simulink model "Mpc_SimMechanics_with_standing"  (R2017b)
settings: Solver=ode45  StartTime=0  StopTime=10  FixedStep=0.0005  EnableMultiTasking=on
InitFcn:
  | isSim = 1;
  | 
  | PreFunctions.CustomInitFcn_with_standing;
  | PreFunctions.simulationInitFcn_with_standing;
undefined symbols (not defined in the file): alpha_x, alpha_y, DiagnosticCodes, DynamicMatrixLibrary, motorPositions, motorVelocities, pelvisPosition, pelvisVelocity, sample_time, X, Y, Z
libraries: sm_lib x170, nesl_utility x75, Contact_Forces_Lib x6, ComponentLibrary x5, xpcrtudplib x2, slrtlib x1
(part 1 of 8)
settings Model: TunableVars=c_CovPos_abduction,c_CovPos_knee,c_CovPos_qj1,c_CovPos_qj2,c_CovPos_qj3,c_CovPos_rotation,c_CovPos_thigh,c_CovPos_toe,c_CovVel_abduction,c_CovVel_knee,c_CovVel_qj1,c_CovVel_qj2,c_CovVel_qj3,c_CovVel_rotation,c_CovVel_thigh,c_CovVel_toe,c_Cov_AngularVelocity,c_Cov_Euler,c_Cov_Euler_rates,c_Cov_LinearAccelerator_xy,c_Cov_LinearAccelerator_z,c_Cov_Lx_LRToe_stTD0,c_Cov_Ly_LRToe_stTD0,c_Cov_Orientation,c_Cov_rpx_LRToe_body,c_Cov_rpx_LRToe_stTD0,c_Cov_rpy_LRToe_body,c_Cov_rpy_LRToe_stTD0,c_Cov_rpz_LRToe_body,c_H_fil_param,c_IK_max_iter_num,c_Kd_abduction,c_Kd_knee,c_Kd_pitch,c_Kd_roll,c_Kd_rotation,c_Kd_st_rotation,c_Kd_thigh,c_Kd_toe,c_Kd_yaw,c_Kp_abduction,c_Kp_knee,c_Kp_pitch,c_Kp_roll,c_Kp_rotation,c_Kp_st_rotation,c_Kp_thigh,c_Kp_toe,c_Kp_yaw,c_KsL_1,c_KsL_2,c_KsR_1,c_KsR_2,c_Tx_slide_toe_2,c_Ty_slide_toe_2,c_Tz_slide_toe_2,c_Vx_tgd_fil_param,c_Vx_tgd_offset,c_Vy_tgd_avg_fil_param,c_Vy_tgd_offset,c_adjusted_desired_roll_angle_fil_param,c_com_x_offset,c_desired_com2stToe_lateral_fil_param,c_dop,c_history_length,c_knee_cp_time,c_lateral_correction_gain,c_max_st_rotation_motor_torque,c_max_turn_per_sec,c_one_step_max_vel_gain,c_rp_LRToe_fil_param,c_st_rotation_torque_ramp_time,c_stance_thre_lb,c_stance_thre_lb_2,c_stance_thre_ub,c_stance_thre_ub_2,c_toe_leave_ground_lb,c_toe_leave_ground_ub,c_torque_transition_time,c_u_abduction_swing_cp,c_u_knee_cp,c_u_pitch_cp,c_u_roll_cp,c_use_dq_AR_for_PD,c_vx_slide_toe_1,c_vx_slide_toe_2,c_vy_slide_toe_1,c_vy_slide_toe_2,c_vz_slide_toe_1,c_vz_slide_toe_2,c_yaw_error_fil_param  TunableVarsStorageClass=Auto,Auto,Auto,Auto,Auto,Auto,Auto,Auto,Auto,Auto,Auto,Auto,Auto,Auto,Auto,Auto,Auto,Auto,Auto,Auto,Auto,Auto,Auto,Auto,Auto,Auto,Auto,Auto,Auto,Auto,Auto,Auto,Auto,Auto,Auto,Auto,Auto,Auto,Auto,Auto,Auto,Auto,Auto,Auto,Auto,Auto,Auto,Auto,Auto,Auto,Auto,Auto,Auto,Auto,Auto,Auto,Auto,Auto,Auto,Auto,Auto,Auto,Auto,Auto,Auto,Auto,Auto,Auto,Auto,Auto,Auto,Auto,Auto,Auto,Auto,Auto,Auto,Auto,Auto,Auto,Auto,Auto,Auto,Auto,Auto,Auto,Auto,Auto,Auto,Auto,Auto  TunableVarsTypeQualifier=,,,,,,,,,,,,,,,,,,,,,,,,,,,,,,,,,,,,,,,,,,,,,,,,,,,,,,,,,,,,,,,,,,,,,,,,,,,,,,,,,,,,,,,,,,  Creator=case  LastModifiedBy=gibso
settings SolverCC: ZeroCrossControl=DisableAll  InsertRTBMode=Always
settings DataIOCC: SaveOutput=off  SignalLogging=off  DSMLogging=off  SaveTime=off
settings OptimizationCC: UseFloatMulNetSlope=on  EfficientFloat2IntCast=on  LifeSpan=inf  SimCompilerOptimization=on  AccelVerboseBuild=on
settings DebuggingCC: ReadBeforeWriteMsg=DisableAll  WriteAfterWriteMsg=DisableAll  WriteAfterReadMsg=DisableAll  ParameterUnderflowMsg=error  ParameterTunabilityLossMsg=error  UniqueDataStoreMsg=error  AllowSymbolicDim=off  StrictBusMsg=ErrorOnBusTreatedAsVector  SFUnexpectedBacktrackingDiag=warning  SFNoUnconditionalDefaultTransitionDiag=warning  SFExecutionAtInitializationDiag=none
settings HardwareCC: TargetBitPerPointer=64  TargetBitPerSizeT=64  TargetBitPerPtrDiffT=64  TargetLongLongMode=on  TargetIntDivRoundTo=Zero  TargetEndianess=LittleEndian  TargetWordSize=64  TargetHWDeviceType=MATLAB Host  ProdEqTarget=off
settings ModelReferenceCC: EnableParallelModelReferenceBuilds=on  ModelReferenceNumInstancesAllowed=Zero  ModelReferenceMinAlgLoopOccurrences=on  PropagateSignalLabelsOutOfModel=off
settings SFSimCC: SimUserIncludeDirs=$root_dir$\CustomCodes\utils\funcs\KinDyn200511_221619
settings SFSimCC: SimUserSources=|
  | R_LeftAbductionJoint_src.c
  | R_LeftThighJoint_src.c
  | R_RightAbductionJoint_src.c
  | R_RightThighJoint_src.c
  | 
  | AMworld_about_pA_src.c
  | 
  | Jb_BasePosX_src.c
  | Jb_BasePosY_src.c
  | Jb_BasePosZ_src.c
  | Jb_BaseRotX_src.c
  | Jb_BaseRotY_src.c
  | Jb_BaseRotZ_src.c
  | Jb_LeftAbductionJoint_src.c
  | Jb_LeftAnkleJoint_src.c
  | Jb_LeftHip_src.c
  | Jb_LeftKneeJoint_src.c
  | Jb_LeftKneeSpringJoint_src.c
  | Jb_LeftKnee_src.c
  | Jb_LeftPelvisRotation_src.c
  | Jb_LeftRotationJoint_src.c
  | Jb_LeftShin_src.c
  | Jb_LeftTarsus_src.c
  | Jb_LeftThighJoint_src.c
  | Jb_LeftThigh_src.c
  | Jb_LeftToeBottomBack_src.c
  | Jb_LeftToeBottomFront_src.c
  | Jb_LeftToeBottom_src.c
  | Jb_LeftToeJoint_src.c
  | Jb_LeftToe_src.c
  | Jb_Pelvis_src.c
  | Jb_RightAbductionJoint_src.c
  | Jb_RightAnkleJoint_src.c
  | Jb_RightHip_src.c
  | Jb_RightKneeJoint_src.c
  | Jb_RightKneeSpringJoint_src.c
  | Jb_RightKnee_src.c
  | Jb_RightPelvisRotation_src.c
  | Jb_RightRotationJoint_src.c
  | Jb_RightShin_src.c
  | Jb_RightTarsus_src.c
  | Jb_RightThighJoint_src.c
  | Jb_RightThigh_src.c
  | Jb_RightToeBottomBack_src.c
  | Jb_RightToeBottomFront_src.c
  | Jb_RightToeBottom_src.c
  | Jb_RightToeJoint_src.c
  | Jb_RightToe_src.c
  | 
  | Jdq_AMworld_about_pA_src.c
  | 
  | 
  | Jp_COM_src.c
  | Jp_LeftAbductionJoint_src.c
  | Jp_LeftAnkleJoint_src.c
  | Jp_LeftHip_src.c
  | Jp_LeftKneeJoint_src.c
  | Jp_LeftKneeSpringJoint_src.c
  | Jp_LeftKnee_src.c
  | Jp_LeftPelvisRotation_src.c
  | Jp_LeftRotationJoint_src.c
  | Jp_LeftShin_src.c
  | Jp_LeftTarsus_src.c
  | Jp_LeftThighJoint_src.c
  | Jp_LeftThigh_src.c
  | Jp_LeftToeBottomBack_src.c
  | Jp_LeftToeBottomFront_src.c
  | Jp_LeftToeBottom_src.c
  | Jp_LeftToeJoint_src.c
  | Jp_LeftToe_src.c
  | Jp_Pelvis_src.c
  | Jp_RightAbductionJoint_src.c
  | Jp_RightAnkleJoint_src.c
  | Jp_RightHip_src.c
  | Jp_RightKneeJoint_src.c
  | Jp_RightKneeSpringJoint_src.c
  | Jp_RightKnee_src.c
  | Jp_RightPelvisRotation_src.c
  | Jp_RightRotationJoint_src.c
  | Jp_RightShin_src.c
  | Jp_RightTarsus_src.c
  | Jp_RightThighJoint_src.c
  | Jp_RightThigh_src.c
  | Jp_RightToeBottomBack_src.c
  | Jp_RightToeBottomFront_src.c
  | Jp_RightToeBottom_src.c
  | Jp_RightToeJoint_src.c
  | Jp_RightToe_src.c
  | 
  | p_BasePosX_src.c
  | p_BasePosY_src.c
  | p_BasePosZ_src.c
  | p_BaseRotX_src.c
  | p_BaseRotY_src.c
  | p_BaseRotZ_src.c
  | p_COM_src.c
  | p_LeftAbductionJoint_src.c
  | p_LeftAnkleJoint_src.c
  | p_LeftHip_src.c
  | p_LeftKneeJoint_src.c
  | p_LeftKneeSpringJoint_src.c
  | p_LeftKnee_src.c
  | p_LeftPelvisRotation_src.c
  | p_LeftRotationJoint_src.c
  | p_LeftShin_src.c
  | p_LeftTarsus_src.c
  | p_LeftThighJoint_src.c
  | p_LeftThigh_src.c
  | p_LeftToeBottomBack_src.c
  | p_LeftToeBottomFront_src.c
  | p_LeftToeBottom_src.c
  | p_LeftToeJoint_src.c
  | p_LeftToe_src.c
  | p_Pelvis_src.c
  | p_RightAbductionJoint_src.c
  | p_RightAnkleJoint_src.c
  | p_RightHip_src.c
  | p_RightKneeJoint_src.c
  | p_RightKneeSpringJoint_src.c
  | p_RightKnee_src.c
  | p_RightPelvisRotation_src.c
  | p_RightRotationJoint_src.c
  | p_RightShin_src.c
  | p_RightTarsus_src.c
  | p_RightThighJoint_src.c
  | p_RightThigh_src.c
  | p_RightToeBottomBack_src.c
  | p_RightToeBottomFront_src.c
  | p_RightToeBottom_src.c
  | p_RightToeJoint_src.c
  | p_RightToe_src.c
  | 
  | T_LeftToeBottomBack_src.c
  | T_LeftToeBottomFront_src.c
  | T_LeftToeBottom_src.c
  | T_RightToeBottomBack_src.c
  | T_RightToeBottomFront_src.c
  | T_RightToeBottom_src.c
  | 
  | J_LL_Left_src.c
  | J_LL_Right_src.c
  | LL_Left_src.c
  | LL_Right_src.c
settings RTWCC: Description=Generic Real-Time Target  RTWUseSimCustomCode=on  CustomInclude=$root_dir$\CustomCodes\utils\funcs\KinDyn200511_221619  BuildConfiguration=Faster Runs  CheckMdlBeforeBuild=Warning
settings RTWCC: CustomSource=|
  | R_LeftAbductionJoint_src.c
  | R_LeftThighJoint_src.c
  | R_RightAbductionJoint_src.c
  | R_RightThighJoint_src.c
  | 
  | AMworld_about_pA_src.c
  | 
  | Jb_BasePosX_src.c
  | Jb_BasePosY_src.c
  | Jb_BasePosZ_src.c
  | Jb_BaseRotX_src.c
  | Jb_BaseRotY_src.c
  | Jb_BaseRotZ_src.c
  | Jb_LeftAbductionJoint_src.c
  | Jb_LeftAnkleJoint_src.c
  | Jb_LeftHip_src.c
  | Jb_LeftKneeJoint_src.c
  | Jb_LeftKneeSpringJoint_src.c
  | Jb_LeftKnee_src.c
  | Jb_LeftPelvisRotation_src.c
  | Jb_LeftRotationJoint_src.c
  | Jb_LeftShin_src.c
  | Jb_LeftTarsus_src.c
  | Jb_LeftThighJoint_src.c
  | Jb_LeftThigh_src.c
  | Jb_LeftToeBottomBack_src.c
  | Jb_LeftToeBottomFront_src.c
  | Jb_LeftToeBottom_src.c
  | Jb_LeftToeJoint_src.c
  | Jb_LeftToe_src.c
  | Jb_Pelvis_src.c
  | Jb_RightAbductionJoint_src.c
  | Jb_RightAnkleJoint_src.c
  | Jb_RightHip_src.c
  | Jb_RightKneeJoint_src.c
  | Jb_RightKneeSpringJoint_src.c
  | Jb_RightKnee_src.c
  | Jb_RightPelvisRotation_src.c
  | Jb_RightRotationJoint_src.c
  | Jb_RightShin_src.c
  | Jb_RightTarsus_src.c
  | Jb_RightThighJoint_src.c
  | Jb_RightThigh_src.c
  | Jb_RightToeBottomBack_src.c
  | Jb_RightToeBottomFront_src.c
  | Jb_RightToeBottom_src.c
  | Jb_RightToeJoint_src.c
  | Jb_RightToe_src.c
  | 
  | Jdq_AMworld_about_pA_src.c
  | 
  | 
  | Jp_COM_src.c
  | Jp_LeftAbductionJoint_src.c
  | Jp_LeftAnkleJoint_src.c
  | Jp_LeftHip_src.c
  | Jp_LeftKneeJoint_src.c
  | Jp_LeftKneeSpringJoint_src.c
  | Jp_LeftKnee_src.c
  | Jp_LeftPelvisRotation_src.c
  | Jp_LeftRotationJoint_src.c
  | Jp_LeftShin_src.c
  | Jp_LeftTarsus_src.c
  | Jp_LeftThighJoint_src.c
  | Jp_LeftThigh_src.c
  | Jp_LeftToeBottomBack_src.c
  | Jp_LeftToeBottomFront_src.c
  | Jp_LeftToeBottom_src.c
  | Jp_LeftToeJoint_src.c
  | Jp_LeftToe_src.c
  | Jp_Pelvis_src.c
  | Jp_RightAbductionJoint_src.c
  | Jp_RightAnkleJoint_src.c
  | Jp_RightHip_src.c
  | Jp_RightKneeJoint_src.c
  | Jp_RightKneeSpringJoint_src.c
  | Jp_RightKnee_src.c
  | Jp_RightPelvisRotation_src.c
  | Jp_RightRotationJoint_src.c
  | Jp_RightShin_src.c
  | Jp_RightTarsus_src.c
  | Jp_RightThighJoint_src.c
  | Jp_RightThigh_src.c
  | Jp_RightToeBottomBack_src.c
  | Jp_RightToeBottomFront_src.c
  | Jp_RightToeBottom_src.c
  | Jp_RightToeJoint_src.c
  | Jp_RightToe_src.c
  | 
  | p_BasePosX_src.c
  | p_BasePosY_src.c
  | p_BasePosZ_src.c
  | p_BaseRotX_src.c
  | p_BaseRotY_src.c
  | p_BaseRotZ_src.c
  | p_COM_src.c
  | p_LeftAbductionJoint_src.c
  | p_LeftAnkleJoint_src.c
  | p_LeftHip_src.c
  | p_LeftKneeJoint_src.c
  | p_LeftKneeSpringJoint_src.c
  | p_LeftKnee_src.c
  | p_LeftPelvisRotation_src.c
  | p_LeftRotationJoint_src.c
  | p_LeftShin_src.c
  | p_LeftTarsus_src.c
  | p_LeftThighJoint_src.c
  | p_LeftThigh_src.c
  | p_LeftToeBottomBack_src.c
  | p_LeftToeBottomFront_src.c
  | p_LeftToeBottom_src.c
  | p_LeftToeJoint_src.c
  | p_LeftToe_src.c
  | p_Pelvis_src.c
  | p_RightAbductionJoint_src.c
  | p_RightAnkleJoint_src.c
  | p_RightHip_src.c
  | p_RightKneeJoint_src.c
  | p_RightKneeSpringJoint_src.c
  | p_RightKnee_src.c
  | p_RightPelvisRotation_src.c
  | p_RightRotationJoint_src.c
  | p_RightShin_src.c
  | p_RightTarsus_src.c
  | p_RightThighJoint_src.c
  | p_RightThigh_src.c
  | p_RightToeBottomBack_src.c
  | p_RightToeBottomFront_src.c
  | p_RightToeBottom_src.c
  | p_RightToeJoint_src.c
  | p_RightToe_src.c
  | 
  | T_LeftToeBottomBack_src.c
  | T_LeftToeBottomFront_src.c
  | T_LeftToeBottom_src.c
  | T_RightToeBottomBack_src.c
  | T_RightToeBottomFront_src.c
  | T_RightToeBottom_src.c
  | 
  | J_LL_Left_src.c
  | J_LL_Right_src.c
  | LL_Left_src.c
  | LL_Right_src.c
settings CodeAppCC: GenerateComments=off  SimulinkBlockComments=off
settings GRTTargetCC: MatFileLogging=off  MultiInstanceERTCode=on  CodeInterfacePackaging=Reusable function  SupportNonFinite=off  GenerateAllocFcn=on
settings ConfigComp: CovMetricSettings=dw  CovHtmlReporting=on  CovSaveCumulativeToWorkspaceVar=on  CovSaveSingleToWorkspaceVar=on  CovExternalEMLEnable=off
settings SimscapeCC: SimscapeNormalizeSystem=off
settings DiagnosticsConfigSet: SimMechanicsRigidlyBoundBlock=warning
settings ExplorerConfigSet: InternalSimMechanicsExplorerSettings="<ExplorerConfiguration><canonicalview>default</canonicalview><AnimationSetting><BasePlaybackSpeed>1.0</BasePlaybackSpeed><PlaybackSpeedFactor>1.0</PlaybackSpeedFactor></AnimationSetting><TilePanel><TileInfo><Tiles Columns=\"1\" Count=\"2\" Rows=\"2\"><Column Weight=\"1\"/><Row Weight=\"0.4993\"/><Row Weight=\"0.5007\"/><Tile Height=\"1\" Width=\"1\" X=\"0\" Y=\"0\"/><Tile Height=\"1\" Width=\"1\" X=\"0\" Y=\"1\"/></Tiles></TileInfo><SceneInfo><SceneViewer><BGColor><R>0.60000002384185791</R><G>0.60000002384185791</G><B>0.60000002384185791</B></BGColor><Camera><DoPerspective>off</DoPerspective><Position><X>35.4589435267912592</X><Y>10.7098035623800421</Y><Z>2.09856989778365666</Z></Position><Center><X>1.22559782766984426e-06</X><Y>10.7098035623800421</Y><Z>2.09856989778365666</Z></Center><Up><X>-0</X><Y>0</Y><Z>1</Z></Up><ViewLimDist>1</ViewLimDist><YLim>6.75206365413680487</YLim><XLim>15.8384121715609041</XLim></Camera></SceneViewer><SceneViewer><BGColor><R>0.60000002384185791</R><G>0.60000002384185791</G><B>0.60000002384185791</B></BGColor><Camera><DoPerspective>off</DoPerspective><Position><X>-0.287232906465883953</X><Y>-35.4589435232020875</Y><Z>0.354651545256036704</Z></Position><Center><X>-0.287232906465883953</X><Y>3.60980493385731904e-07</Y><Z>0.354651545256036704</Z></Center><Up><X>0</X><Y>-0</Y><Z>1</Z></Up><ViewLimDist>1</ViewLimDist><YLim>2.45492732079823162</YLim><XLim>5.74215193839130489</XLim></Camera></SceneViewer></SceneInfo></TilePanel><MechEditorPanel><Cameras><Camera><Id>Camera1</Id><Value><Name>Tracking Camera</Name><NativeCamera><PositionTrackingFeature>Cassie.Cassie_Simulation.World.Tracking_Camera.F</PositionTrackingFeature><CenterTrackingFeature>Cassie.Cassie_Simulation.World.Tracking_Camera_Target.F</CenterTrackingFeature><UpVectorTrackingFeature>Cassie.Cassie_Simulation.World.Tracking_Camera_Target.F</UpVectorTrackingFeature><CenterTrackingOrigin>on</CenterTrackingOrigin><UpVectorTrackingDirection>+Z</UpVectorTrackingDirection></NativeCamera></Value></Camera><Camera><Id>Camera2</Id><Value><Name>Fixed Camera</Name><NativeCamera><PositionTrackingFeature>Cassie.Cassie_Simulation.World.Fixed_Camera.F</PositionTrackingFeature><CenterTrackingFeature>Cassie.Cassie_Simulation.World.Fixed_Camera_Target.F</CenterTrackingFeature><UpVectorTrackingFeature>Cassie.Cassie_Simulation.World.Fixed_Camera_Target.F</UpVectorTrackingFeature><CenterTrackingOrigin>on</CenterTrackingOrigin><UpVectorTrackingDirection>+Z</UpVectorTrackingDirection></NativeCamera></Value></Camera><Camera><Id>Camera3</Id><Value><Name>tracking camera positive y</Name><NativeCamera><PositionTrackingFeature>Cassie.Cassie_Simulation.Cassie_Pelvis_World</PositionTrackingFeature><CenterTrackingFeature/><UpVectorTrackingFeature/><CenterTrackingOrigin>off</CenterTrackingOrigin><CenterTrackingDirection>+Y</CenterTrackingDirection><UpVectorTrackingDirection>+Z</UpVectorTrackingDirection></NativeCamera></Value></Camera></Cameras><GfxPanelCameraMap/><VideoCreator><PlaybackSpeedRatio>1.0</PlaybackSpeedRatio><FrameRate>30</FrameRate><VideoFormat>MPEG-4</VideoFormat><FrameSize>[1920 1080]</FrameSize></VideoCreator></MechEditorPanel></ExplorerConfiguration>"

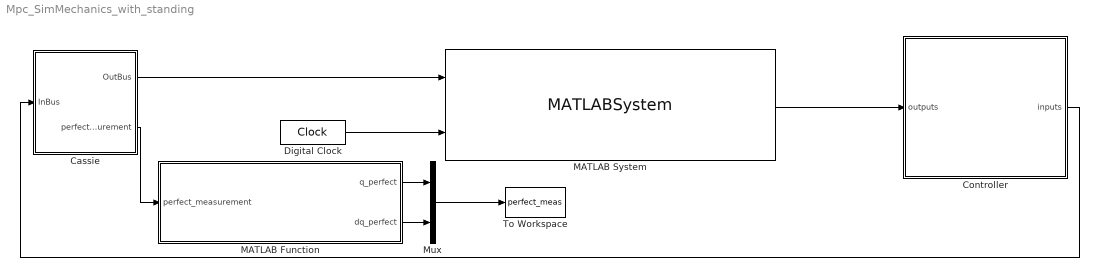
== system Mpc_SimMechanics_with_standing ==
  Cassie : Subsystem  InitFcn=|  StartFcn=|  StopFcn=|
      InitFcn=|
      | % Start clock at initialization (used for computing real time performance)
      | initTime = tic;
      | 
      | % Import bus definitions
      | CassieModule.importBuses;
      StartFcn=|
      | % Store build time
      | buildTime = toc(initTime);
      StopFcn=|
      | % Store computation time
      | computationTime = toc(initTime) - buildTime;
      | 
      | % Get simulation time
      | simulationTime = get_param(bdroot, 'SimulationTime');
      | 
      | % Compute real time performance
      | percentRealTime = 100*simulationTime/computationTime;
      | 
      | % Display
      | fprintf('Build time: %0.2f seconds \n', buildTime);
      | fprintf('Simulation time: %0.2f seconds \n', simulationTime);
      | fprintf('Computation time: %0.2f seconds \n', computationTime);
      | fprintf('Performance: %0.2f%% real time \n', percentRealTime);
      mask Display: image('Cassie.png');
  Controller : Subsystem
  Digital Clock : DigitalClock  SampleTime=sample_time
  MATLAB Function : MATLAB Function  TreatAsAtomicUnit=on
  MATLAB System : MATLABSystem  System=RemoteSpoofer_with_standing  SimulateUsing=Code generation
      mask Type: RemoteSpoofer_with_standing
      mask Display:
      | disp('RemoteSpoofer_with_standing');
      | port_label('input',1,'cassieOutputs');
      | port_label('input',2,'t');
      | port_label('output',1,'cassieOutputs');
  Mux : Mux  Inputs=2
  To Workspace : ToWorkspace  VariableName=perfect_meas  SaveFormat=Timeseries  SampleTime=-1
  wires:
  Cassie/1(OutBus) -> MATLAB System/1
  Digital Clock/1 -> MATLAB System/2
  MATLAB System/1 -> Controller/1(outputs)
  Controller/1("inputs ") -> Cassie/1(InBus)
  Cassie/2(perfect measurement) -> MATLAB Function/1(perfect_measurement)
  MATLAB Function/1(q_perfect) -> Mux/1
  MATLAB Function/2(dq_perfect) -> Mux/2
  Mux/1 -> To Workspace/1

== system Mpc_SimMechanics_with_standing/Cassie ==
  InBus : Inport
  Cassie Core MATLAB System : MATLABSystem  System=CassieCoreSim  SimulateUsing=Code generation
      mask Type: CassieCoreSim
      mask Display: disp('CassieCoreSim');
  Cassie Simulation : Subsystem
      mask Display: image('Cassie.png');
  Delay : Delay  DelayLength=1
  Rate Transition : RateTransition  OutPortSampleTime=0.0005
  Signal Conversion : SignalConversion  ConversionOutput=Nonvirtual bus  OutDataTypeStr=Bus: CassieOutBus  OverrideOpt=off
  OutBus : Outport  OutDataTypeStr=Bus: CassieOutBus
  perfect measurement : Outport  Port=2
  wires:
  Signal Conversion/1 -> Cassie Core MATLAB System/2, OutBus/1
  Cassie Simulation/1(OutBus) -> Rate Transition/1
  Rate Transition/1 -> Signal Conversion/1
  Delay/1 -> Cassie Simulation/1(InBus)
  Cassie Core MATLAB System/1 -> Delay/1
  InBus/1 -> Cassie Core MATLAB System/1
  Cassie Simulation/2(perfect measurement) -> perfect measurement/1

== system Mpc_SimMechanics_with_standing/Controller ==
  outputs : Inport  OutDataTypeStr=Bus: CassieOutBus
  Bus Assignment : BusAssignment  AssignedSignals=dq
  Constant : Constant  Value=isSim  OutDataTypeStr=int8  LockScale=on
  Constant1 : Constant  Value=DynamicMatrixLibrary  OutDataTypeStr=Bus: cassieDynamicMatrixLibraryBus
  Delay : Delay  DelayLength=1  InitialCondition=0
  Digital Clock : DigitalClock  SampleTime=sample_time
  MATLAB Function1 : MATLAB Function  TreatAsAtomicUnit=on
  MATLAB System : MATLABSystem  System=RadioCommandInterpreter_with_standing  max_turn_per_sec=c_max_turn_per_sec  Vx_tgd_fil_param=c_Vx_tgd_fil_param  Vy_tgd_avg_fil_param=c_Vy_tgd_avg_fil_param  H_fil_param=c_H_fil_param  desired_com2stToe_lateral_fil_param=c_desired_com2stToe_lateral_fil_param  yaw_stand_filter_param=c_yaw_stand_filter_param  pitch_stand_filter_param=c_pitch_stand_filter_param  roll_stand_filter_param=c_roll_stand_filter_param  p_com_stand_y_filter_param=c_p_com_stand_y_filter_param  sample_time=sample_time  SimulateUsing=Code generation
      mask Type: RadioCommandInterpreter_with_standing
      mask Display:
      | disp('RadioCommandInterpreter_with_standing');
      | port_label('input',1,'cassieOutputs');
      | port_label('output',1,'IRC');
  MATLAB System2 : MATLABSystem  System=PolyRegressionFilter_2  sample_time=sample_time  history_length=c_history_length  dop=c_dop  signal_dim=20  delay=0  max_history_length=20  max_dop=3  SimulateUsing=Code generation
      mask Type: PolyRegressionFilter_2
      mask Display:
      | disp('PolyRegressionFilter_2');
      | port_label('input',1,'q');
      | port_label('output',1,'dq');
  MATLAB System4 : MATLABSystem  System=StateEstimator_with_standing  Ks_L1=c_KsL_1  Ks_L2=c_KsL_2  Ks_R1=c_KsR_1  Ks_R2=c_KsR_2  Cov_LRT_r_body_x=c_Cov_rpx_LRToe_body  Cov_LRT_r_body_y=c_Cov_rpy_LRToe_body  Cov_LRT_r_body_z=c_Cov_rpz_LRToe_body  Cov_LinearAccelerator_xy=c_Cov_LinearAccelerator_xy  Cov_LinearAccelerator_z=c_Cov_LinearAccelerator_z  vx_slide_toe_1=c_vx_slide_toe_1  vx_slide_toe_2=c_vx_slide_toe_2  Tx_slide_toe_2=c_Tx_slide_toe_2  vy_slide_toe_1=c_vy_slide_toe_1  vy_slide_toe_2=c_vy_slide_toe_2  Ty_slide_toe_2=c_Ty_slide_toe_2  vz_slide_toe_1=c_vz_slide_toe_1  vz_slide_toe_2=c_vz_slide_toe_2  Tz_slide_toe_2=c_Tz_slide_toe_2  sample_time=sample_time  SimulateUsing=Code generation
      mask Type: StateEstimator_with_standing
      mask Display:
      | disp('StateEstimator_with_standing');
      | port_label('input',1,'cassieOutputs');
      | port_label('input',2,'IRC');
      | port_label('input',3,'t_total');
      | port_label('input',4,'isSim');
      | port_label('input',5,'Controller2Estimator');
      | port_label('output',1,'EstStates');
      | port_label('output',2,'q');
      | port_label('output',3,'EulerRates');
      | port_label('output',4,'q_xyz');
      | port_label('output',5,'dq_xyz');
      | port_label('output',6,'a_world');
  MATLAB System6 : MATLABSystem  System=Cassie_MPC_With_Standing  Kp_pitch=c_Kp_pitch  Kd_pitch=c_Kd_pitch  Kp_roll=c_Kp_roll  Kd_roll=c_Kd_roll  Kp_yaw=c_Kp_yaw  Kd_yaw=c_Kd_yaw  Kp_abduction=c_Kp_abduction  Kp_rotation=c_Kp_rotation  Kp_thigh=c_Kp_thigh  Kp_knee=c_Kp_knee  Kp_toe=c_Kp_toe  Kd_abduction=c_Kd_abduction  Kd_rotation=c_Kd_rotation  Kd_thigh=c_Kd_thigh  Kd_knee=c_Kd_knee  Kd_toe=c_Kd_toe  Kp_st_rotation=c_Kp_st_rotation  Kd_st_rotation=c_Kd_st_rotation  u_abduction_swing_cp=c_u_abduction_swing_cp  u_roll_cp=c_u_roll_cp  u_pitch_cp=c_u_pitch_cp  u_knee_cp=c_u_knee_cp  CovPos_abduction=c_CovPos_abduction  CovPos_rotation=c_CovPos_rotation  CovPos_thigh=c_CovPos_thigh  CovPos_knee=c_CovPos_knee  CovPos_toe=c_CovPos_toe  CovPos_qj1=c_CovPos_qj1  CovPos_qj2=c_CovPos_qj2  CovPos_qj3=c_CovPos_qj3  CovVel_abduction=c_CovVel_abduction  CovVel_rotation=c_CovVel_rotation  CovVel_thigh=c_CovVel_thigh  CovVel_knee=c_CovVel_knee  CovVel_toe=c_CovVel_toe  CovVel_qj1=c_CovVel_qj1  CovVel_qj2=c_CovVel_qj2  CovVel_qj3=c_CovVel_qj3  Cov_Euler=c_Cov_Euler  Cov_Euler_rates=c_Cov_Euler_rates  Cov_Lx_LRToe_stTD0=c_Cov_Lx_LRToe_stTD0  Cov_Ly_LRToe_stTD0=c_Cov_Ly_LRToe_stTD0  Cov_rpx_LRToe_stTD0=c_Cov_rpx_LRToe_stTD0  Cov_rpy_LRToe_stTD0=c_Cov_rpy_LRToe_stTD0  torque_transition_time=c_torque_transition_time  knee_cp_time=c_knee_cp_time  st_rotation_torque_ramp_time=c_st_rotation_torque_ramp_time  torque_standFromWalk_transition_time=c_torque_standFromWalk_transition_time  com_x_offset=c_com_x_offset  Vx_tgd_offset=c_Vx_tgd_offset  Vy_tgd_offset=c_Vy_tgd_offset  stance_thre_lb=c_stance_thre_lb  stance_thre_ub=c_stance_thre_ub  stance_thre_lb_2=c_stance_thre_lb_2  stance_thre_ub_2=c_stance_thre_ub_2  IK_max_iter_num=c_IK_max_iter_num  yaw_error_fil_param=c_yaw_error_fil_param  rp_LRToe_fil_param=c_rp_LRToe_fil_param  adjusted_desired_roll_angle_fil_param=c_adjusted_desired_roll_angle_fil_param  use_dq_AR_for_PD=c_use_dq_AR_for_PD  lateral_correction_gain=c_lateral_correction_gain  one_step_max_vel_gain=c_one_step_max_vel_gain  max_st_rotation_motor_torque=c_max_st_rotation_motor_torque  KsL_1=c_KsL_1  KsL_2=c_KsL_2  KsR_1=c_KsR_1  KsR_2=c_KsR_2  toe_leave_ground_lb=c_toe_leave_ground_lb  toe_leave_ground_ub=c_toe_leave_ground_ub  Kp_abduction_stand=c_Kp_abduction_stand  Kp_rotation_stand=c_Kp_rotation_stand  Kp_thigh_stand=c_Kp_thigh_stand  Kp_knee_stand=c_Kp_knee_stand  Kp_toe_stand=c_Kp_toe_stand  Kd_abduction_stand=c_Kd_abduction_stand  Kd_rotation_stand=c_Kd_rotation_stand  Kd_thigh_stand=c_Kd_thigh_stand  Kd_knee_stand=c_Kd_knee_stand  Kd_toe_stand=c_Kd_toe_stand  Kp_knee_stand_lateral=c_Kp_knee_stand_lateral  Kd_knee_stand_lateral=c_Kd_knee_stand_lateral  com_x_offset_stand=c_com_x_offset_stand  F_st_lb_stand=c_F_st_lb_stand  F_st_ub_stand=c_F_st_ub_stand  com_y_offset_stand2walk=c_com_y_offset_stand2walk  last_width_walk2stand=c_last_width_walk2stand  V_com_x_offset_walk2stand=c_V_com_x_offset_walk2stand  mu_fil_param=c_mu_fil_param  sample_time=sample_time  SimulateUsing=Interpreted execution
      mask Type: Cassie_MPC_With_Standing
      mask Display:
      | disp('Cassie_MPC_With_Standing');
      | port_label('input',1,'LinuxToSlrt');
      | port_label('input',2,'Est_States_Bus');
      | port_label('input',3,'t_total');
      | port_label('input',4,'isSim');
      | port_label('input',5,'IRC');
      | port_label('input',6,'DynamicMatrixLibrary');
      | port_label('output',1,'userInputs');
      | port_label('output',2,'Data');
      | port_label('output',3,'SlrtToLinux');
      | port_label('output',4,'Controller2Estimator');
  Rate Transition2 : RateTransition  OutPortSampleTime=sample_time
  Rate Transition4 : RateTransition  OutPortSampleTime=sample_time
  To Workspace : ToWorkspace  VariableName=Data  SaveFormat=Timeseries  SampleTime=-1
  To Workspace2 : ToWorkspace  VariableName=EstStates  SaveFormat=Timeseries  SampleTime=-1
  To Workspace3 : ToWorkspace  VariableName=EulerRates  SaveFormat=Timeseries  SampleTime=-1
  To Workspace4 : ToWorkspace  VariableName=qxyz  SaveFormat=Timeseries  SampleTime=-1
  To Workspace5 : ToWorkspace  VariableName=dqxyz  SaveFormat=Timeseries  SampleTime=-1
  To Workspace7 : ToWorkspace  VariableName=a_world  SaveFormat=Timeseries  SampleTime=-1
  file_scopes : Subsystem  Commented=on
  mpc_lip_footplacement : Subsystem
  scopes : Subsystem  Commented=on
  "inputs " : Outport  OutDataTypeStr=Bus: CassieUserInBus
  wires:
  MATLAB System4/6 -> To Workspace7/1
  Digital Clock/1 -> MATLAB System6/3, MATLAB System4/3
  Constant/1 -> MATLAB System6/4, MATLAB System4/4
  outputs/1 -> Rate Transition4/1
  Constant1/1 -> MATLAB System6/6
  MATLAB System6/1 -> "inputs "/1
  Rate Transition4/1 -> MATLAB System/1, MATLAB System4/1
  MATLAB Function1/1(dq) -> Bus Assignment/2
  MATLAB System2/1 -> MATLAB Function1/1("dq ")
  MATLAB System4/1 -> Rate Transition2/1
  MATLAB System/1 -> MATLAB System6/5, MATLAB System4/2
  Rate Transition2/1 -> Bus Assignment/1
  MATLAB System6/2 -> file_scopes/1(In1), scopes/1(In1), To Workspace/1
  Bus Assignment/1 -> MATLAB System6/2, To Workspace2/1
  mpc_lip_footplacement/1("LinuxToSlrt ") -> MATLAB System6/1
  MATLAB System6/3 -> mpc_lip_footplacement/1(SlrtToLinux)
  MATLAB System4/4 -> To Workspace4/1
  MATLAB System4/5 -> MATLAB Function1/2(dqxyz), To Workspace5/1
  MATLAB System4/3 -> MATLAB Function1/3(EulerRates), To Workspace3/1
  MATLAB System4/2 -> MATLAB System2/1
  MATLAB System6/4 -> Delay/1
  Delay/1 -> MATLAB System4/5
